simulink model "Suspensao_Passiva"  (Simulink 7.6)
settings: Solver=ode45  StartTime=0.0  StopTime=10.0  RelTol=1e-3
libraries: simulink x1
settings Model: Creator=Reginaldo Cardoso  LastModifiedBy=Reginaldo Cardoso
settings DebuggingCC: SolverPrmCheckMsg=none
settings GRTTargetCC: CombineOutputUpdateFcns=on

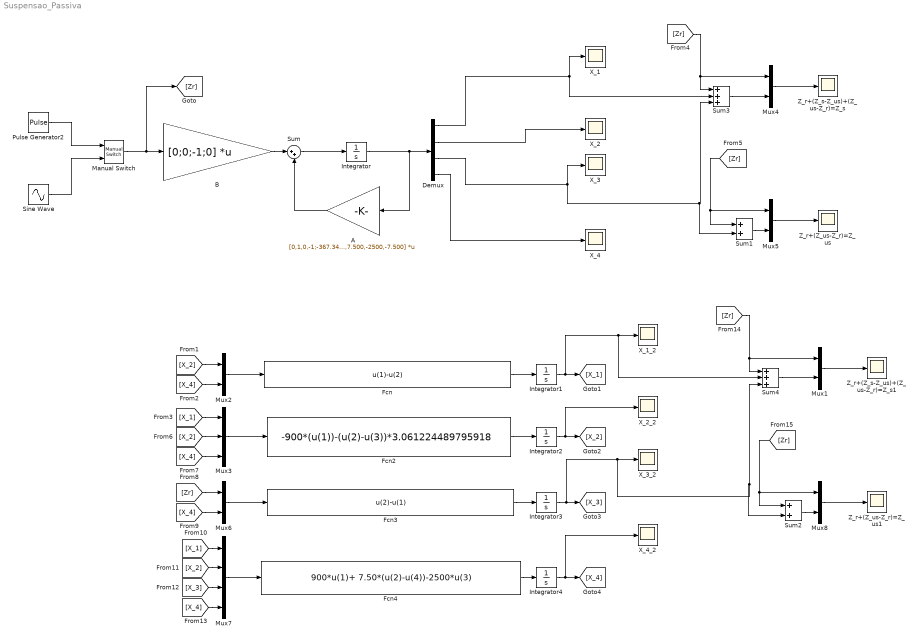
== system Suspensao_Passiva ==
  A : Gain  Gain=[0,1,0,-1;-367.3469,-3.061224489795918,0,3.061224489795918;0,0,0,1;900,7.500,-2500,-7.500]  Multiplication=Matrix(K*u) (u vector)
  B : Gain  Gain=[0;0;-1;0]  Multiplication=Matrix(K*u)
  Demux : Demux
  Fcn : Fcn  Expr=u(1)-u(2)
  Fcn2 : Fcn  Expr=-900*(u(1))-(u(2)-u(3))*3.061224489795918
  Fcn3 : Fcn  Expr=u(2)-u(1)
  Fcn4 : Fcn  Expr=900*u(1)+ 7.50*(u(2)-u(4))-2500*u(3)
  Integrator{,1..4} (5 alike) : Integrator
  Manual Switch : simulink/Signal Routing/Manual Switch  SystemSampleTime=-1  sw=1  action=0  varsize=off
  Mux{1..2,4..6,8} (6 alike) : Mux  Inputs=2
  Mux3 : Mux  Inputs=3
  Mux7 : Mux
  Pulse Generator2 : DiscretePulseGenerator  PulseType=Time based  Amplitude=0.02  Period=3  PulseWidth=50  PhaseDelay=.1
  Sine Wave : Sin  Amplitude=0.02  Frequency=pi/0.3  SampleTime=0
  Sum : Sum  Inputs=|++
  Sum1 : Sum  Inputs=2  SaturateOnIntegerOverflow=on  InputSameDT=on  OutDataTypeStr=Inherit: Same as first input
  Sum2 : Sum  Inputs=2  SaturateOnIntegerOverflow=on  InputSameDT=on  OutDataTypeStr=Inherit: Same as first input
  Sum3 : Sum  Inputs=3  SaturateOnIntegerOverflow=on  InputSameDT=on  OutDataTypeStr=Inherit: Same as first input
  Sum4 : Sum  Inputs=3  SaturateOnIntegerOverflow=on  InputSameDT=on  OutDataTypeStr=Inherit: Same as first input
  X_{1..4} (4 alike) : Scope
      X_1 settings: SaveName=x  DataFormat=Array
      X_2 settings: SaveName=x1  DataFormat=Array
      X_3 settings: SaveName=x2  DataFormat=Array
      X_4 settings: SaveName=x3  DataFormat=Array
  X_1_2 : Scope
      settings: SaveName=x6  DataFormat=Array
  "X_2_2 " : Scope
      settings: SaveName=x7  DataFormat=Array
  "X_3_2 " : Scope
      settings: SaveName=x8  DataFormat=Array
  "X_4_2 " : Scope
      settings: SaveName=x9  DataFormat=Array
  Z_r+(Z_s-Z_us)+(Z_us-Z_r)=Z_s : Scope
      settings: SaveName=x4  DataFormat=Array
  Z_r+(Z_s-Z_us)+(Z_us-Z_r)=Z_s1 : Scope
      settings: SaveName=x10  DataFormat=Array
  Z_r+(Z_us-Z_r)=Z_us : Scope
      settings: SaveName=x5  DataFormat=Array
  Z_r+(Z_us-Z_r)=Z_us1 : Scope
      settings: SaveName=x11  DataFormat=Array
  wires:
  A/1 -> Sum/2
  Sum/1 -> Integrator/1
  B/1 -> Sum/1
  Demux/1 -> X_1/1, Sum3/2
  Demux/3 -> X_3/1, Sum1/2, Sum3/3
  Integrator/1 -> A/1, Demux/1
  Demux/2 -> X_2/1
  Demux/4 -> X_4/1
  [Zr] -> Mux4/1, Sum3/1
  [Zr] -> Mux5/1, Sum1/1
  Sum3/1 -> Mux4/2
  Sum1/1 -> Mux5/2
  Mux5/1 -> Z_r+(Z_us-Z_r)=Z_us/1
  Mux4/1 -> Z_r+(Z_s-Z_us)+(Z_us-Z_r)=Z_s/1
  Sine Wave/1 -> Manual Switch/2
  Pulse Generator2/1 -> Manual Switch/1
  Manual Switch/1 -> B/1, [Zr]
  Mux2/1 -> Fcn/1
  Mux3/1 -> Fcn2/1
  Mux6/1 -> Fcn3/1
  Mux7/1 -> Fcn4/1
  [X_2] -> Mux2/1
  [X_4] -> Mux2/2
  [X_1] -> Mux3/1
  [X_2] -> Mux3/2
  [X_4] -> Mux3/3
  [Zr] -> Mux6/1
  [X_4] -> Mux6/2
  [X_1] -> Mux7/1
  [X_2] -> Mux7/2
  [X_3] -> Mux7/3
  [X_4] -> Mux7/4
  Fcn/1 -> Integrator1/1
  Fcn2/1 -> Integrator2/1
  Fcn3/1 -> Integrator3/1
  Fcn4/1 -> Integrator4/1
  Integrator4/1 -> "X_4_2 "/1, [X_4]
  Integrator2/1 -> "X_2_2 "/1, [X_2]
  Integrator1/1 -> Sum4/2, X_1_2/1, [X_1]
  Integrator3/1 -> Sum2/2, Sum4/3, "X_3_2 "/1, [X_3]
  [Zr] -> Mux1/1, Sum4/1
  [Zr] -> Mux8/1, Sum2/1
  Sum4/1 -> Mux1/2
  Sum2/1 -> Mux8/2
  Mux8/1 -> Z_r+(Z_us-Z_r)=Z_us1/1
  Mux1/1 -> Z_r+(Z_s-Z_us)+(Z_us-Z_r)=Z_s1/1
